simulink model "BESS"  (R2024b)
settings: Solver=VariableStepAuto  StartTime=0  StopTime=400  FixedStep=1  MaxStep=1e-5  RelTol=1e-3
undefined symbols (not defined in the file or in its folder): Ion, Lithium
libraries: spsSeriesRLCBranchLib x3, spsBatteryLib x1, spsDiodeLib x1, spsIGBTDiodeLib x1, spsPWMGeneratorDCDCLib x1, spsMultimeterLib x1, spsPVArrayLib x1, spsSeriesRLCLoadLib x1, sps_lib x1
settings Model: Creator=mitphanase  LastModifiedBy=mitphanase
settings SolverCC: EnableFixedStepZeroCrossing=on

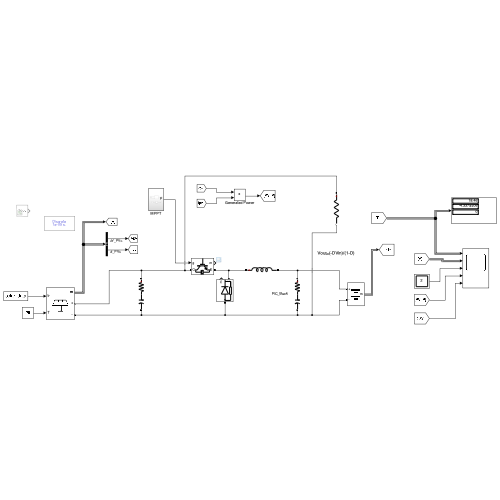
[thumbnail: Simulink's stored preview of the top-level diagram]
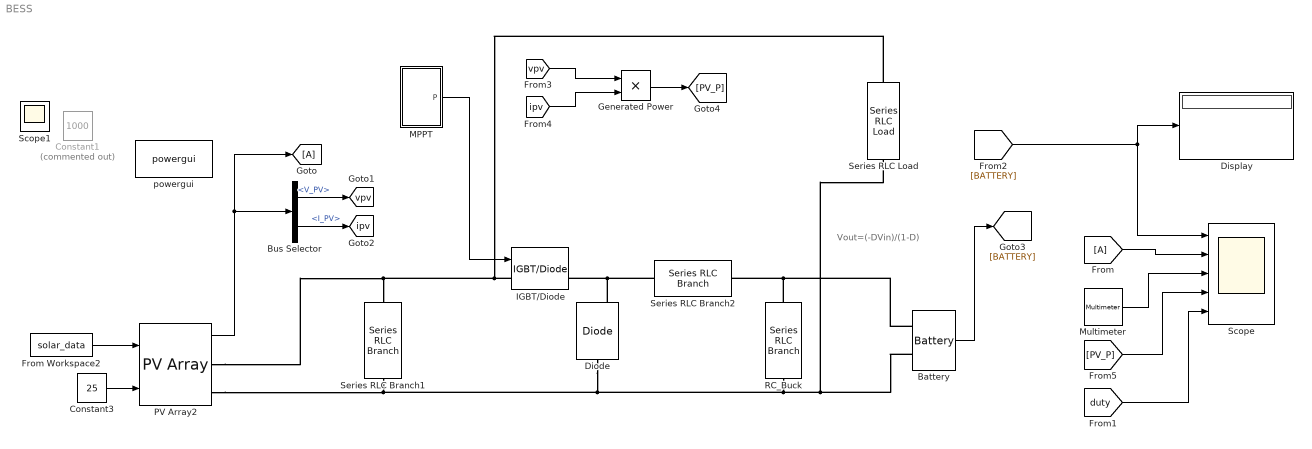
== system BESS ==
  note: Vout=(-DVin)/(1-D)
  Battery : spsBatteryLib/Battery  BatType=Lithium-Ion  NomV=400  NomQ=31.25  SOC=10  Batt_Tr=1  PresetModel=on  MaxQ=31.25  MinV=300  FullV=465.5949  Dis_rate=13.587  R=0.128  Normal_OP=28.2609  expZone="[432.1543      1.535326]"
  Bus Selector : BusSelector  OutputSignals=V_PV,I_PV
  Constant1 : Constant  Commented=on  Value=1000
  Constant3 : Constant  Value=25
  Diode : spsDiodeLib/Diode  Ron=0.001  Lon=0  Vf=0.8  IC=0  UseSnubber=0  Rs=500  Cs=250e-9  Measurements=on
  Display : Display
  From : From
  From Workspace2 : FromWorkspace  VariableName=solar_data  OutDataTypeStr=double  SampleTime=1
  Generated Power : Product
  Goto : Goto
  IGBT/Diode : spsIGBTDiodeLib/IGBT//Diode  Ron=1e-3  Rs=1e5  Cs=inf  Measurements=on
  MPPT : Subsystem
  Multimeter : spsMultimeterLib/Multimeter  L=4  sel=[2 4]  yselected={}  Gain=[1 1]  OutputType=Complex  PlotAtSimulationStop=off  PhasorSimulation=off
  PV Array2 : spsPVArrayLib/PV Array  Npar=4  Nser=7  PlotType=array @ 1000 W/m2 & specified temperatures  S_vec="[ 1000  500  100 ]"  Temp_C_vec="[ 45 25  ]"  ModuleName=SunPower SPR-415E-WHT-D  PlotWhenSelected=off  Pm=414.801  Ncell=128  Voc=85.3  Isc=6.09  Vm=72.9  Im=5.69  beta_Voc_pc=-0.229  alpha_Isc_pc=0.030706  beta_Voc=-0.19534  alpha_Isc=0.00187  IL=6.0978  I0=7.1698e-13  nI=0.87223  Rsh=419.7781  Rs=0.53711  RobustModel=off  RobustCellTemperature=313.3991  BAL=on  Tc=1e-6  Tfilter=5e-5
  RC_Buck : spsSeriesRLCBranchLib/Series RLC Branch  LConnTagsString=__new0  RConnTagsString=__new0  BranchType=RC  Resistance=1e-4  Inductance=1e-3  SetiL0=off  InitialCurrent=0  Capacitance=3300e-6  Setx0=off  InitialVoltage=24  Measurements=Branch voltage and current
  Scope : Scope  NumInputPorts=5
  Series RLC Branch1 : spsSeriesRLCBranchLib/Series RLC Branch  LConnTagsString=__new0  RConnTagsString=__new0  BranchType=RC  Resistance=1e-4  Inductance=1e-3  SetiL0=off  InitialCurrent=0  Capacitance=10000e-6  Setx0=off  InitialVoltage=0  Measurements=Branch voltage
  Series RLC Branch2 : spsSeriesRLCBranchLib/Series RLC Branch  LConnTagsString=__new0  RConnTagsString=__new0  BranchType=L  Resistance=0.1  Inductance=0.8653e-3  SetiL0=off  InitialCurrent=0  Capacitance=1e-6  Setx0=off  InitialVoltage=0  Measurements=Branch current
  Series RLC Load : spsSeriesRLCLoadLib/Series RLC Load  LConnTagsString=a  RConnTagsString=__new0  NominalVoltage=400  NominalFrequency=60  ActivePower=10e3  InductivePower=0  CapacitivePower=0  Setx0=off  InitialVoltage=0  SetiL0=off  InitialCurrent=0  Measurements=None  LoadType=constant Z
  powergui : sps_lib/powergui  Priority=1  SimulationMode=Discrete  SampleTime=10e-6  frequency=60  Iterations=50  frequencyindice=0  Pbase=100e6  ErrMax=1e-4  UnitsV=kV  UnitsW=MW  buscounter=0  FunctionMessages=off  echomessages=off  EnableUseOfTLC=off  CurrentSourceSwitches=off  DisableSnubberDevices=off  DisableRonSwitches=off  DisableVfSwitches=off  DisplayEquations=off  AutomaticDiscreteSolvers=off  SolverType=Tustin/Backward Euler (TBE)  Interpol=off  ExternalGateDelay=off  methode=off  Ts=100  x0status=blocks  SPID=on  SwTol=0  HookPort=off  NonlinearTolerance=1e-4  nMaxIteration=100  ContinueOnMaxIteration=off  RestoreLinks=warning  ResistiveCurrentMeasurement=off  Frange=[0:2:500]  Ylog=off  Xlog=on  ShowGrid=off  save=off  variable=ZData  structure=0  ZoomFFT=off  StartTime=0.0  cycles=1  DisplayStyle=1  fundamental=60  FreqAxis=off  MaxFrequency=1000  frequencyindicesteady=1  RmsSteady=1  display=off
  Scope1 : Scope
  tag scope: ipv=global, vpv=global
  wires:
  PV Array2/1 -> Goto/1, Bus Selector/1
  From/1 -> Scope/2
  Constant3/1 -> PV Array2/2
  Bus Selector/1 -> [vpv]  "<V_PV>"
  Bus Selector/2 -> [ipv]  "<I_PV>"
  Battery/1 -> [BATTERY]
  [BATTERY] -> Scope/1, Display/1
  [vpv] -> Generated Power/1
  [ipv] -> Generated Power/2
  Generated Power/1 -> [PV_P]
  From Workspace2/1 -> PV Array2/1
  Multimeter/1 -> Scope/3
  [PV_P] -> Scope/4
  [duty] -> Scope/5
  MPPT/1(P) -> IGBT/Diode/1
  connections:
  Series RLC Branch1/RConn1 -- PV Array2/RConn2 -- Series RLC Load/RConn1 -- Battery/LConn2 -- RC_Buck/RConn1 -- Diode/LConn1
  RC_Buck/LConn1 -- Battery/LConn1 -- Series RLC Branch2/RConn1
  PV Array2/RConn1 -- Series RLC Load/LConn1 -- IGBT/Diode/LConn1 -- Series RLC Branch1/LConn1
  Diode/RConn1 -- Series RLC Branch2/LConn1 -- IGBT/Diode/RConn1

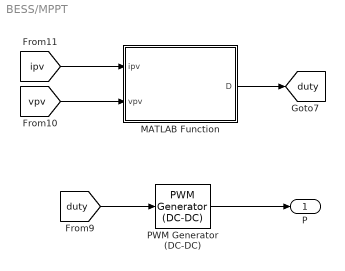
== system BESS/MPPT ==
  MATLAB Function : MATLAB Function  TreatAsAtomicUnit=on
  PWM Generator (DC-DC) : spsPWMGeneratorDCDCLib/PWM Generator (DC-DC)  Fsw=5000  Ts=0
  P : Outport
  tag scope: duty=global
  wires:
  [duty] -> PWM Generator (DC-DC)/1
  MATLAB Function/1(D) -> [duty]
  PWM Generator (DC-DC)/1 -> P/1
  [ipv] -> MATLAB Function/1(ipv)
  [vpv] -> MATLAB Function/2(vpv)

== matlab function BESS/MPPT/MATLAB Function ==
  data: ipv input; D output; vpv input
function D = pno_mppt(ipv, vpv)
        % P&O MPPT algorithm for PV system (optimized for buck converter)
        % Inputs: ipv - PV current (A), vpv - PV voltage (V)
        % Output: D - Duty cycle (0.1 to 0.9)

        persistent P_prev V_prev D_prev;
        if isempty(P_prev)
            P_prev = 0;
            V_prev = 0;
            D_prev = 0.5;
        end

        delta_D = 0.005;
        D_min = 0.1;
        D_max = 0.9;

        if isnan(ipv) || isnan(vpv) || ipv < 0 || vpv < 0
            D = D_prev;
            return;
        end

        P = ipv * vpv;
        delta_P = P - P_prev;
        delta_V = vpv - V_prev;

        if delta_P > 0
            if delta_V > 0
                D = D_prev + delta_D; % Increase voltage (increase D for buck)
            else
                D = D_prev - delta_D; % Decrease voltage (decrease D)
            end
        else
            if delta_V > 0
                D = D_prev - delta_D; % Decrease voltage (decrease D)
            else
                D = D_prev + delta_D; % Increase voltage (increase D)
            end
        end

        D = min(D_max, max(D_min, D));
        P_prev = P;
        V_prev = vpv;
        D_prev = D;
    end
